simulink model "FB_Controller_SIM"  (R2025b)
settings: Solver=FixedStepDiscrete  StartTime=0.0  StopTime=tspan  FixedStep=dt_sim  RelTol=rel_tol  AbsTol=abs_tol
undefined symbols (not defined in the file): Cimub, const_voltage, dt_data, use_true_state_flag
libraries: mspsensorlib x1
settings Model: Creator=koryh  LastModifiedBy=koryh

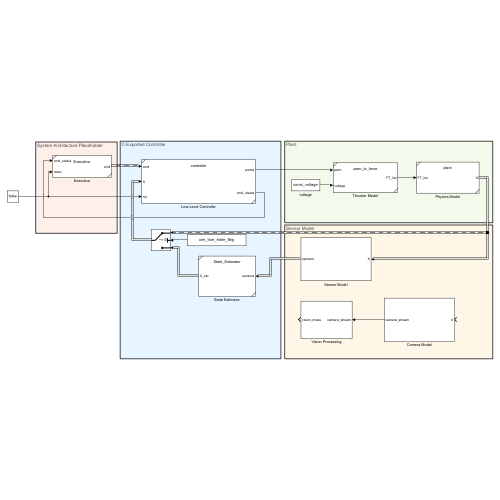
[thumbnail: Simulink's stored preview of the top-level diagram]
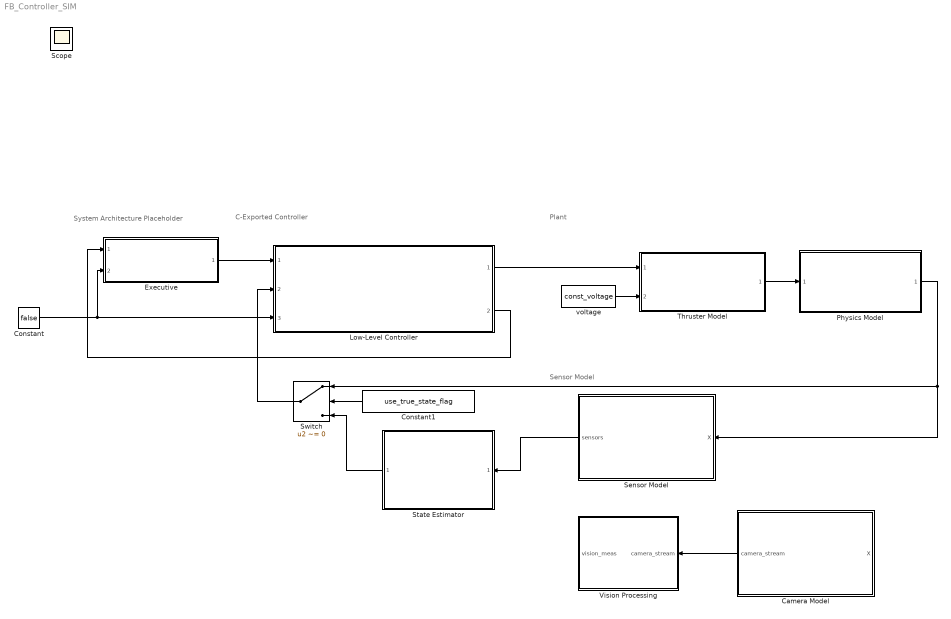
== system FB_Controller_SIM ==
  note: System Architecture Placeholder
  note: Sensor Model
  note: Plant
  note: C-Exported Controller
  Camera Model : Subsystem
  Constant : Constant  Value=false
  Constant1 : Constant  Value=use_true_state_flag
  Executive : Subsystem  ReferencedSubsystem=Executive
  Low-Level Controller : Subsystem  ReferencedSubsystem=controller
  Physics Model : Subsystem  ReferencedSubsystem=plant
  Sensor Model : Subsystem
  State Estimator : Subsystem  ReferencedSubsystem=State_Estimator
  Switch : Switch  Criteria=u2 ~= 0  SaturateOnIntegerOverflow=off  InputSameDT=off
  Thruster Model : Subsystem  ReferencedSubsystem=pwm_to_force
  Vision Processing : Subsystem
  voltage : Constant  Value=const_voltage
  Scope : Scope
      settings: ActiveDisplayYMinimum=-0.048832566475369238  ActiveDisplayYMaximum=0.79721663606048965
  wires:
  voltage/1 -> Thruster Model/2
  Low-Level Controller/1 -> Thruster Model/1
  Thruster Model/1 -> Physics Model/1
  Executive/1 -> Low-Level Controller/1
  Low-Level Controller/2 -> Executive/1
  Physics Model/1 -> Sensor Model/1(X), Switch/1
  Camera Model/1(camera_stream) -> Vision Processing/1(camera_stream)
  Sensor Model/1(sensors) -> State Estimator/1
  Constant/1 -> Executive/2, Low-Level Controller/3
  Switch/1 -> Low-Level Controller/2
  Constant1/1 -> Switch/2
  State Estimator/1 -> Switch/3

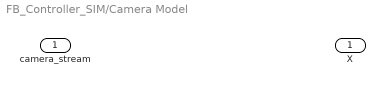
== system FB_Controller_SIM/Camera Model ==
  X : Inport
  camera_stream : Outport

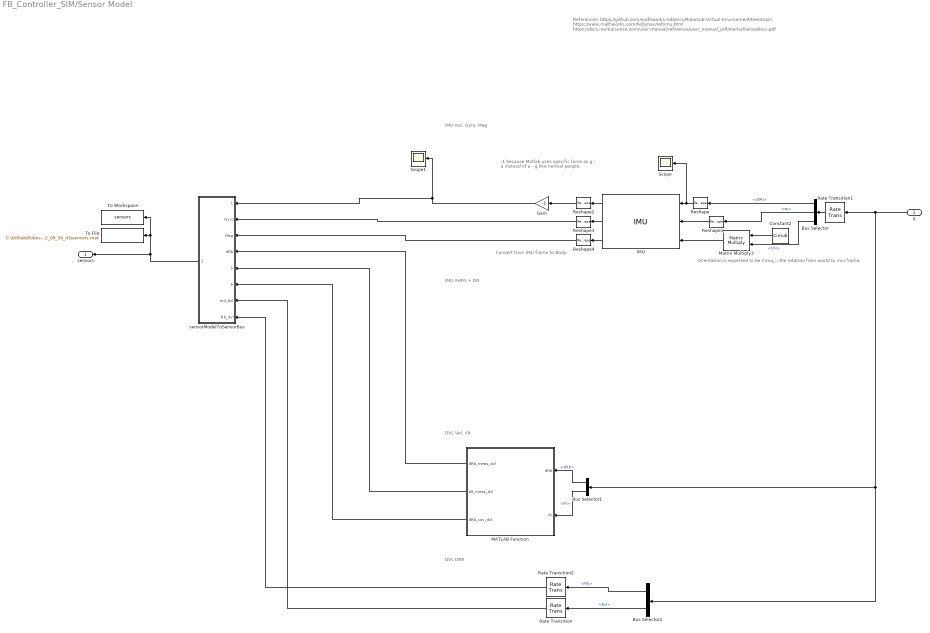
== system FB_Controller_SIM/Sensor Model ==
  note: DVL DRR
  note: IMU AHRS + DR
  note: IMU Acc, Gyro, Mag
  note: -1 because Matlab uses specific force as
      |  g - a instead of a - g like normal people.
  note: Orientation is expected to be Cimu_i, the rotation from world to imu frame.
  note: Convert from IMU frame to Body
  note: References:
      | https://github.com/mathworks-robotics/RoboSub-Virtual-Environment/tree/main
      | https://www.mathworks.com/help/nav/ref/imu.html
      | https://docs.inertialsense.com/user-manual/reference/user_manual_pdf/InertialSenseDocs.pdf
  note: DVL Vel, Alt
  X : Inport  OutDataTypeStr=Bus: X_bus
  Bus Selector : BusSelector  OutputSignals=ddRi,wi,Cbi
  Bus Selector1 : BusSelector  OutputSignals=dRb,Ri
  Bus Selector2 : BusSelector  OutputSignals=Rb,Eul
  Constant2 : Constant  Value=Cimub
  Gain : Gain  Gain=-1
  IMU : mspsensorlib/IMU  DispRefFrame=NED  TemperaturePort=off  Temperature=imu.T  MagneticFieldPort=off  MagneticFieldNED=imu.Bi  MagneticFieldENU=[ -2.4169, 27.5550, 16.0849 ]  SeedDouble=67  SimulateUsing=Interpreted execution  AccelParamsMeasurementRange=imu.acc.meas_range  AccelParamsResolution=imu.acc.res  AccelParamsConstantBias=imu.acc.const_bias  AccelParamsAxesMisalignment=imu.acc.axes_skew  AccelParamsNoiseDensity=imu.acc.vel_rand_walk  AccelParamsBiasInstability=imu.acc.bias_inst  AccelParamsBiasInstabilityNumerator=imu.acc.bias_inst_num_coeffs  AccelParamsBiasInstabilityDenominator=imu.acc.bias_inst_den_coeffs  AccelParamsRandomWalk=imu.acc.acc_rand_walk  AccelParamsNoiseType=double-sided  AccelParamsTemperatureBias=imu.acc.temp_bias  AccelParamsTemperatureScaleFactor=imu.acc.temp_scale_factor  GyroParamsMeasurementRange=imu.gyro.max_read  GyroParamsResolution=imu.gyro.res  GyroParamsConstantBias=imu.gyro.const_bias  GyroParamsAxesMisalignment=imu.gyro.axes_skew  GyroParamsAccelerationBias=imu.gyro.bias_from_acc  GyroParamsNoiseDensity=imu.gyro.angle_rand_walk  GyroParamsBiasInstability=imu.gyro.bias_inst  GyroParamsBiasInstabilityNumerator=imu.gyro.bias_inst_filter_num_coeffs  GyroParamsBiasInstabilityDenominator=imu.gyro.bias_inst_filter_den_coeffs  GyroParamsRandomWalk=imu.gyro.rate_rand_walk  GyroParamsNoiseType=double-sided  GyroParamsTemperatureBias=imu.gyro.temp_bias  GyroParamsTemperatureScaleFactor=imu.gyro.temp_scale_factor  MagParamsMeasurementRange=imu.mag.max_read  MagParamsResolution=imu.mag.res  MagParamsConstantBias=imu.mag.const_bias  MagParamsAxesMisalignment=imu.mag.axes_skew  MagParamsNoiseDensity=imu.mag.white_noise_psd  MagParamsBiasInstability=imu.mag.bias_inst  MagParamsBiasInstabilityNumerator=imu.mag.bias_inst_filter_num_coeffs  MagParamsBiasInstabilityDenominator=imu.mag.bias_isnt_filter_den_coeffs  MagParamsRandomWalk=imu.mag.rand_walk  MagParamsNoiseType=double-sided  MagParamsTemperatureBias=imu.mag.temp_bias  MagParamsTemperatureScaleFactor=imu.mag.temp_scale_factor
  MATLAB Function : MATLAB Function  TreatAsAtomicUnit=on
  Matrix Multiply3 : Product  Multiplication=Matrix(*)
  Rate Transition : RateTransition  OutPortSampleTime=dt_dvl
  Rate Transition1 : RateTransition  OutPortSampleTime=dt_imu
  Rate Transition2 : RateTransition  OutPortSampleTime=dt_dvl
  Reshape : Reshape  OutputDimensionality=Row vector (2-D)
  Reshape1 : Reshape  OutputDimensionality=Row vector (2-D)
  Reshape2 : Reshape  OutputDimensionality=Column vector (2-D)
  Reshape3 : Reshape  OutputDimensionality=Column vector (2-D)
  Reshape4 : Reshape  OutputDimensionality=Column vector (2-D)
  Scope : Scope
      settings: ActiveDisplayYMinimum=-1  ActiveDisplayYMaximum=1
  Scope1 : Scope
      settings: ActiveDisplayYMinimum=-1  ActiveDisplayYMaximum=1  DataLoggingVariableName=ScopeData7
  To File : ToFile  Filename=C:\Github\Robosub\SimulinkPlant\data\2026_05_02_09_56_43\sensors.mat  MatrixName=sensors  SaveFormat=Timeseries
  To Workspace : ToWorkspace  VariableName=sensors  SaveFormat=Timeseries  SampleTime=dt_data
  sensorModelToSensorBus : MATLAB Function  TreatAsAtomicUnit=on
  sensors : Outport  OutDataTypeStr=Bus: sensor_bus
  wires:
  X/1 -> Rate Transition1/1, Bus Selector1/1, Bus Selector2/1
  Reshape/1 -> Scope/1, IMU/1
  Bus Selector/2 -> Reshape1/1  "<wi>"
  IMU/1 -> Reshape2/1
  IMU/2 -> Reshape3/1
  IMU/3 -> Reshape4/1
  Reshape1/1 -> IMU/2
  Bus Selector/1 -> Reshape/1  "<ddRi>"
  Matrix Multiply3/1 -> IMU/3
  Constant2/1 -> Matrix Multiply3/1
  Bus Selector/3 -> Matrix Multiply3/2  "<Cbi>"
  Reshape2/1 -> Gain/1
  Bus Selector1/1 -> MATLAB Function/1(dRb)  "<dRb>"
  Bus Selector1/2 -> MATLAB Function/2(Ri)  "<Ri>"
  Bus Selector2/1 -> Rate Transition2/1  "<Rb>"
  sensorModelToSensorBus/1(sensors) -> To File/1, To Workspace/1, sensors/1
  Gain/1 -> Scope1/1, sensorModelToSensorBus/1(linAccel)
  Reshape3/1 -> sensorModelToSensorBus/2(Gyro)
  Reshape4/1 -> sensorModelToSensorBus/3(Mag)
  MATLAB Function/1(dRb_meas_dvl) -> sensorModelToSensorBus/4(dRb)
  MATLAB Function/2(alt_meas_dvl) -> sensorModelToSensorBus/5(alt_meas_dvl)
  MATLAB Function/3(dRb_cov_dvl) -> sensorModelToSensorBus/6(dRb_cov_dvl)
  Bus Selector2/2 -> Rate Transition/1  "<Eul>"
  Rate Transition/1 -> sensorModelToSensorBus/7(eul_dvl)
  Rate Transition1/1 -> Bus Selector/1
  Rate Transition2/1 -> sensorModelToSensorBus/8(Rb_dvl)

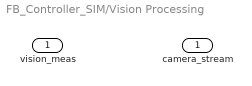
== system FB_Controller_SIM/Vision Processing ==
  camera_stream : Inport
  vision_meas : Outport

== matlab function FB_Controller_SIM/Sensor Model/MATLAB Function ==
  data: dRb input; dRb_meas_dvl output; Ri input; alt_meas_dvl output; dRb_cov_dvl output; dvl parameter
function [dRb_meas_dvl, alt_meas_dvl, dRb_cov_dvl] = dvl_sim(dRb, Ri,dvl)
%{
Model from this repository:
https://github.com/mathworks-robotics/RoboSub-Virtual-Environment/
Need to modify this to give erroneous or no reading when ground lock is
available.

Also need to add noise to the altitude measurement and determine if it
needs modification based on attitude.
%}
%get altitude (assumes Ri is measured from the robot's starting depth
true_depth = dvl.start_depth + Ri(3); 
true_alt = dvl.pool_depth - true_depth;
alt_meas_dvl = true_alt;

%bias for velocity measurements
persistent bias
if isempty(bias)
    bias = zeros(3,1);
end


% ---------------- Update bias (Gauss-Markov) ----------------
if dvl.bias_tau > 0 && dvl.bias_sigma_ss > 0
    % Discrete-time OU: b_{k+1} = (1 - dt/tau) b_k + sqrt(2*sigma^2*dt/tau) * w
    a = max(0.0, 1.0 - dvl.bias_dt/dvl.bias_tau);
    q = sqrt(max(0.0, 2.0*dvl.bias_sigma_ss^2*dvl.bias_dt/dvl.bias_tau));
    bias = a*bias + q * randn(3,1);
else
    bias = zeros(3,1);
end

% ---------------- Add noise & bias ----------------
noise = dvl.noise_sigma .* randn(3,1);    % white noise
dRb_meas_dvl = dRb + bias + noise;

dRb_cov_dvl = diag([dvl.noise_sigma].^2);

== matlab function FB_Controller_SIM/Sensor Model/sensorModelToSensorBus ==
  data: linAccel input; sensors output Bus: sensor_bus; Gyro input; Mag input; dRb input; alt_meas_dvl input; dRb_cov_dvl input; eul_dvl input; Rb_dvl input
function sensors = fcn(linAccel,Gyro,Mag,dRb,alt_meas_dvl,dRb_cov_dvl, eul_dvl, Rb_dvl)

sensors = sensorModelToSensorBus(linAccel,Gyro,Mag,dRb,alt_meas_dvl,dRb_cov_dvl, eul_dvl, Rb_dvl);
